simulink model "computing_speed"  (R2024b)
settings: Solver=FixedStepAuto  StartTime=0.0  StopTime=Tend  FixedStep=Tsim  RelTol=1e-4
values from neighbouring files (symbols this model uses):
  p = 1    [setup.m]
  pole_1_Hz = -10    [computing_speed.m]    (also in setup.m)
  pole_2_Hz = -100    [computing_speed.m]    (also in setup.m)
  speed_cmd = 3000    [setup.m]
settings Model: Creator=puroh  LastModifiedBy=tnoguchi
settings OptimizationCC: DefaultParameterBehavior=Inlined  EnhancedBackFolding=on  PassReuseOutputArgsAs=Individual arguments  ZeroExternalMemoryAtStartup=off  ZeroInternalMemoryAtStartup=off  OptimizeBlockOrder=speed  DifferentSizesBufferReuse=on  EfficientTunableParamExpr=on
settings DebuggingCC: ParameterTunabilityLossMsg=error  UnconnectedInputMsg=warning  UnconnectedOutputMsg=warning  UnconnectedLineMsg=warning
settings ModelReferenceCC: EnableRefExpFcnMdlSchedulingChecks=on
settings SFSimCC: MATLABDynamicMemAlloc=off
settings RTWCC: Description=Embedded Coder  SystemTargetFile=ert.tlc  TemplateMakefile=ert_default_tmf  GPUComputeCapability=3.5  DLArmComputeVersion=19.05
settings CodeAppCC: ForceParamTrailComments=on  IgnoreCustomStorageClasses=off  OperatorAnnotations=on  SimulinkDataObjDesc=on  SFDataObjDesc=on  InsertBlockDesc=on
settings ERTTargetCC: TargetLangStandard=C99 (ISO)  ERTCustomFileTemplate=example_file_process.tlc  DynamicArrayContainerType=coder::array

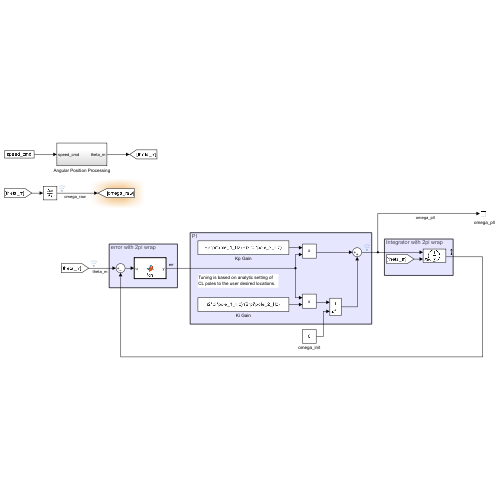
[thumbnail: Simulink's stored preview of the top-level diagram]
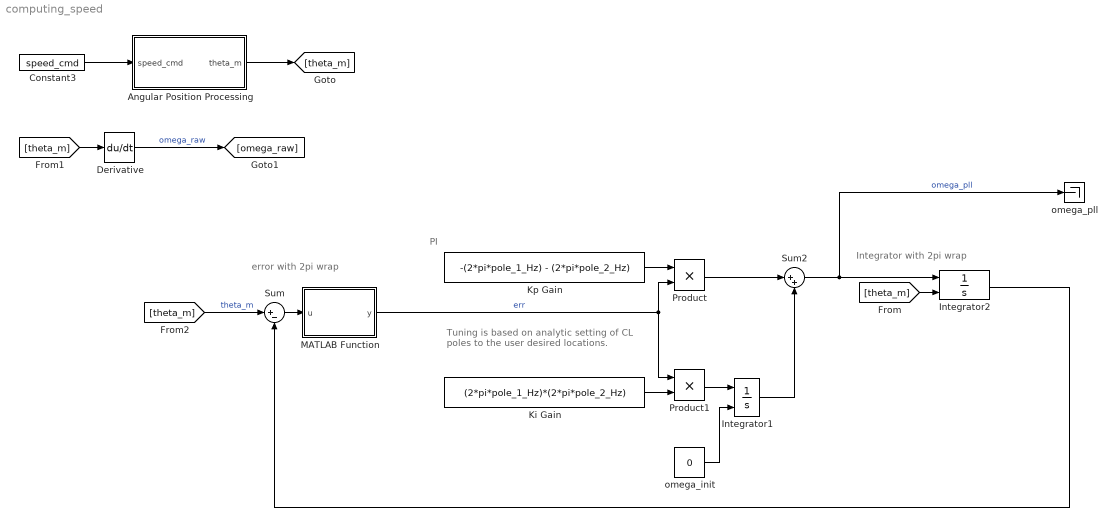
== system computing_speed ==
  note: Integrator with 2pi wrap
  note: error with 2pi wrap
  note: PI
  note: Tuning is based on analytic setting of CL poles to the user desired locations.
  Angular Position Processing : Subsystem
  Constant3 : Constant  Value=speed_cmd
  Derivative : Derivative
  Integrator1 : Integrator  InitialConditionSource=external
  Integrator2 : Integrator  InitialConditionSource=external  WrapState=on
  Ki Gain : Constant  Value=(2*pi*pole_1_Hz)*(2*pi*pole_2_Hz)
  Kp Gain : Constant  Value=-(2*pi*pole_1_Hz) - (2*pi*pole_2_Hz)
  MATLAB Function : MATLAB Function  TreatAsAtomicUnit=on
  Product : Product
  Product1 : Product
  Sum : Sum  Inputs=|+-
  Sum2 : Sum  Inputs=|++
  omega_init : Constant  Value=0
  omega_pll : Terminator
  wires:
  MATLAB Function/1(y) -> Product1/1, Product/2  "err"
  Product/1 -> Sum2/1
  Kp Gain/1 -> Product/1
  Ki Gain/1 -> Product1/2
  Product1/1 -> Integrator1/1
  Integrator1/1 -> Sum2/2
  omega_init/1 -> Integrator1/2
  Sum/1 -> MATLAB Function/1(u)
  Sum2/1 -> omega_pll/1, Integrator2/1  "omega_pll"
  Integrator2/1 -> Sum/2
  [theta_m] -> Integrator2/2
  Constant3/1 -> Angular Position Processing/1(speed_cmd)
  Angular Position Processing/1(theta_m) -> [theta_m]
  [theta_m] -> Derivative/1
  Derivative/1 -> [omega_raw]  "omega_raw"
  [theta_m] -> Sum/1  "theta_m"

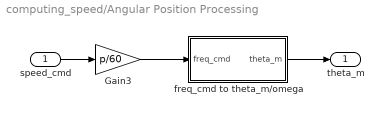
== system computing_speed/Angular Position Processing ==
  speed_cmd : Inport
  Gain3 : Gain  Gain=p/60
  freq_cmd to theta_m/omega : Subsystem
  theta_m : Outport
  wires:
  Gain3/1 -> freq_cmd to theta_m/omega/1(freq_cmd)
  speed_cmd/1 -> Gain3/1
  freq_cmd to theta_m/omega/1(theta_m) -> theta_m/1

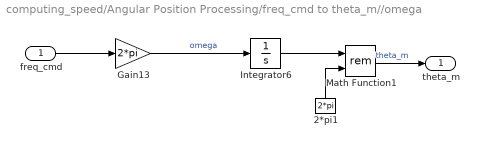
== system computing_speed/Angular Position Processing/freq_cmd to theta_m//omega ==
  freq_cmd : Inport
  2*pi1 : Constant  Value=2*pi
  Gain13 : Gain  Gain=2*pi
  Integrator6 : Integrator
  Math Function1 : Math  Operator=rem  SignedPower=on
  theta_m : Outport
  wires:
  Integrator6/1 -> Math Function1/1
  freq_cmd/1 -> Gain13/1
  2*pi1/1 -> Math Function1/2
  Gain13/1 -> Integrator6/1  "omega"
  Math Function1/1 -> theta_m/1  "theta_m"

== matlab function computing_speed/MATLAB Function ==
  data: u input; y output
function y = fcn(u)

y = u;

if y > pi
    y = y - 2*pi;
end

if y < -pi
    y = y + 2*pi;
end
